simulink model "Combined"  (R2022a)
settings: Solver=FixedStepAuto  StartTime=0.0  StopTime=10.0  FixedStep=1e-3  RelTol=1e-3  EnableMultiTasking=on
undefined symbols (not defined in the file or in its folder): D0, D1, D10, D11, D12, D13, D2, D4, D5, D6, D7, D8, D9, PTA0, PTA2, PTB23, PTB9, PTC16, PTC17, PTC2, PTC3, PTC4, PTD0, PTD1, PTD2, PTD3
libraries: frdmk64flib x14
settings Model: ExtModeTrigDuration=5  Creator=anand  LastModifiedBy=anand
settings OptimizationCC: EnhancedBackFolding=on  PassReuseOutputArgsAs=Individual arguments  ZeroExternalMemoryAtStartup=off  ZeroInternalMemoryAtStartup=off  MaxStackSize=64  OptimizeBlockOrder=speed  DifferentSizesBufferReuse=on  OptimizationCustomize=off  EfficientTunableParamExpr=on
settings DebuggingCC: ParameterTunabilityLossMsg=error
settings HardwareCC: ProdBitPerPointer=32  ProdBitPerSizeT=32  ProdBitPerPtrDiffT=32  ProdLargestAtomicInteger=Long  ProdLargestAtomicFloat=Double  ProdWordSize=32  ProdHWDeviceType=ARM Compatible->ARM Cortex
settings SFSimCC: MATLABDynamicMemAlloc=off
settings RTWCC: SystemTargetFile=ert.tlc  HardwareBoard=NXP FRDM-K64F  TLCOptions="-aInlineSetEventsForThisBaseRateFcn=TLC_FALSE -aSuppressMultiTaskScheduler=TLC_FALSE  -aRateBasedStepFcn=0"  TemplateMakefile=ert_default_tmf  Toolchain=GNU Tools for ARM Embedded Processors
settings CodeAppCC: ForceParamTrailComments=on  IgnoreCustomStorageClasses=off  OperatorAnnotations=on  SimulinkDataObjDesc=on  SFDataObjDesc=on  InsertBlockDesc=on
settings ERTTargetCC: ExtModeTransport=4  ExtModeMexFile=sendToCommService

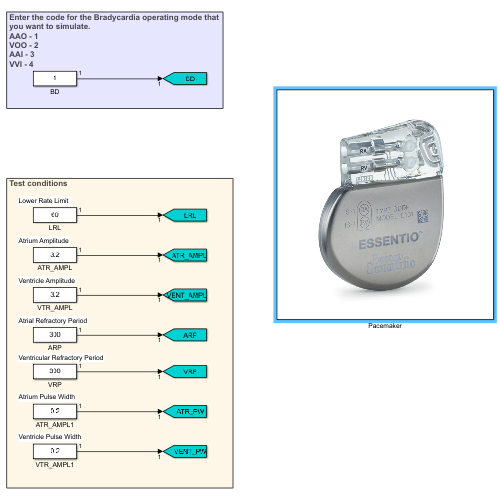
[thumbnail: Simulink's stored preview of the top-level diagram]
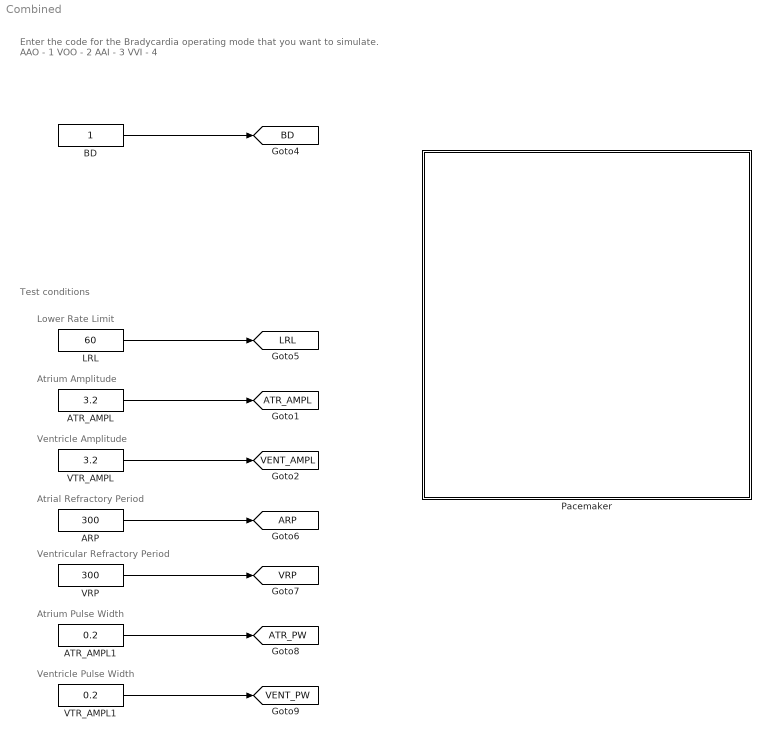
== system Combined ==
  note: Lower Rate Limit
  note: Test conditions
  note: Enter the code for the Bradycardia operating mode that
      | you want to simulate.
      | AAO - 1
      | VOO - 2
      | AAI - 3
      | VVI - 4
  note: Atrium Amplitude
  note: Ventricle Amplitude
  note: Atrial Refractory Period
  note: Ventricular Refractory Period
  note: Atrium Pulse Width
  note: Ventricle Pulse Width
  ARP : Constant  Value=300
  ATR_AMPL : Constant  Value=3.2
  ATR_AMPL1 : Constant  Value=0.2
  BD : Constant
  LRL : Constant  Value=60
  Pacemaker : Subsystem
      mask Display: image('$imagefile'); % Use "Edit Image" on toolstrip to change.
  VRP : Constant  Value=300
  VTR_AMPL : Constant  Value=3.2
  VTR_AMPL1 : Constant  Value=0.2
  tag scope: ARP=global, ATR_AMPL=global, ATR_PW=global, BD=global, LRL=global, VENT_AMPL=global, VENT_PW=global, VRP=global
  wires:
  LRL/1 -> [LRL]
  BD/1 -> [BD]
  ATR_AMPL/1 -> [ATR_AMPL]
  VTR_AMPL/1 -> [VENT_AMPL]
  ARP/1 -> [ARP]
  VRP/1 -> [VRP]
  ATR_AMPL1/1 -> [ATR_PW]
  VTR_AMPL1/1 -> [VENT_PW]

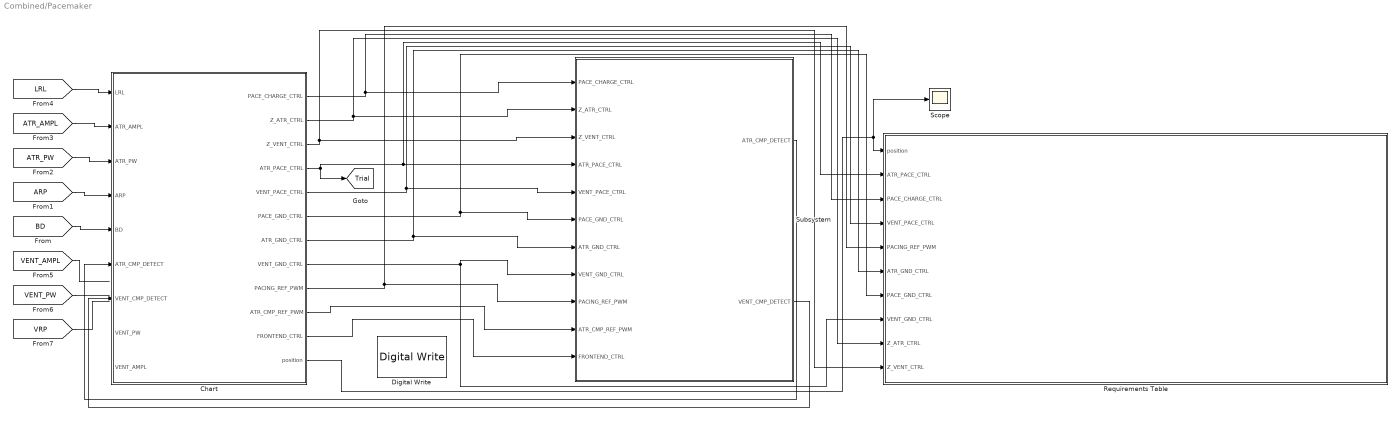
== system Combined/Pacemaker ==
  Chart : Stateflow chart  TreatAsAtomicUnit=on
  Digital Write : frdmk64flib/Digital Write  Whichpin=RED_LED
  Requirements Table : Requirements Table  TreatAsAtomicUnit=on
  Scope : Scope
  Subsystem : Subsystem
  tag scope: Trial=global
  wires:
  Chart/1(PACE_CHARGE_CTRL) -> Requirements Table/3(PACE_CHARGE_CTRL), Subsystem/1(PACE_CHARGE_CTRL)
  Chart/11(FRONTEND_CTRL) -> Subsystem/11(FRONTEND_CTRL)
  Subsystem/1(ATR_CMP_DETECT) -> Chart/6(ATR_CMP_DETECT)
  Chart/2(Z_ATR_CTRL) -> Requirements Table/9(Z_ATR_CTRL), Subsystem/2(Z_ATR_CTRL)
  Chart/6(PACE_GND_CTRL) -> Requirements Table/7(PACE_GND_CTRL), Subsystem/6(PACE_GND_CTRL)
  Chart/3(Z_VENT_CTRL) -> Requirements Table/10(Z_VENT_CTRL), Subsystem/3(Z_VENT_CTRL)
  Chart/9(PACING_REF_PWM) -> Requirements Table/5(PACING_REF_PWM), Subsystem/9(PACING_REF_PWM)
  Chart/8(VENT_GND_CTRL) -> Requirements Table/8(VENT_GND_CTRL), Subsystem/8(VENT_GND_CTRL)
  Chart/10(ATR_CMP_REF_PWM) -> Subsystem/10(ATR_CMP_REF_PWM)
  Chart/7(ATR_GND_CTRL) -> Requirements Table/6(ATR_GND_CTRL), Subsystem/7(ATR_GND_CTRL)
  Chart/5(VENT_PACE_CTRL) -> Requirements Table/4(VENT_PACE_CTRL), Subsystem/5(VENT_PACE_CTRL)
  Chart/4(ATR_PACE_CTRL) -> [Trial], Requirements Table/2(ATR_PACE_CTRL), Subsystem/4(ATR_PACE_CTRL)
  [BD] -> Chart/5(BD)
  [ATR_AMPL] -> Chart/2(ATR_AMPL)
  [ARP] -> Chart/4(ARP)
  [LRL] -> Chart/1(LRL)
  [ATR_PW] -> Chart/3(ATR_PW)
  [VENT_AMPL] -> ?
  [VENT_PW] -> ?
  [VRP] -> ?
  Subsystem/2(VENT_CMP_DETECT) -> Chart/7(VENT_CMP_DETECT)
  Chart/12(position) -> Scope/1, Requirements Table/1(position)

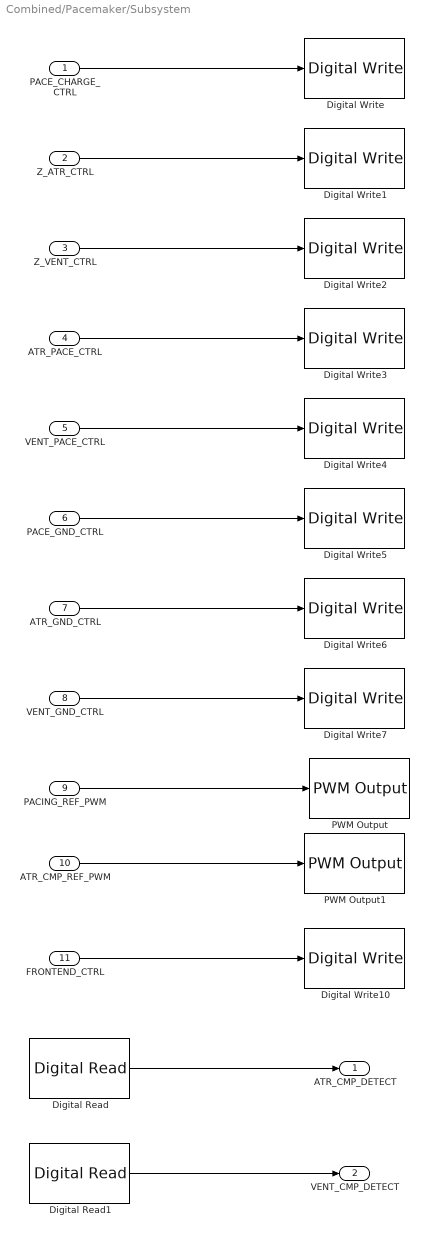
== system Combined/Pacemaker/Subsystem ==
  PACE_CHARGE_CTRL : Inport  OutDataTypeStr=boolean
  Z_ATR_CTRL : Inport  Port=2  OutDataTypeStr=boolean
  Z_VENT_CTRL : Inport  Port=3
  ATR_PACE_CTRL : Inport  Port=4
  VENT_PACE_CTRL : Inport  Port=5
  PACE_GND_CTRL : Inport  Port=6
  ATR_GND_CTRL : Inport  Port=7
  VENT_GND_CTRL : Inport  Port=8
  PACING_REF_PWM : Inport  Port=9
  ATR_CMP_REF_PWM : Inport  Port=10
  FRONTEND_CTRL : Inport  Port=11
  Digital Read : frdmk64flib/Digital Read  Whichpin=PTC16 (D0)  SampleTime=-1
  Digital Read1 : frdmk64flib/Digital Read  Whichpin=PTC17 (D1)  SampleTime=-1
  Digital Write : frdmk64flib/Digital Write  Whichpin=PTB9 (D2)
  Digital Write1 : frdmk64flib/Digital Write  Whichpin=PTB23 (D4)
  Digital Write10 : frdmk64flib/Digital Write  Whichpin=PTD1 (D13)
  Digital Write2 : frdmk64flib/Digital Write  Whichpin=PTC3 (D7)
  Digital Write3 : frdmk64flib/Digital Write  Whichpin=PTA0 (D8)
  Digital Write4 : frdmk64flib/Digital Write  Whichpin=PTC4 (D9)
  Digital Write5 : frdmk64flib/Digital Write  Whichpin=PTD0 (D10)
  Digital Write6 : frdmk64flib/Digital Write  Whichpin=PTD2 (D11)
  Digital Write7 : frdmk64flib/Digital Write  Whichpin=PTD3 (D12)
  PWM Output : frdmk64flib/PWM Output  Whichpin=PTA2 (D5)  InitialFrequency=2000  InitialDutyCycle=0
  PWM Output1 : frdmk64flib/PWM Output  Whichpin=PTC2 (D6)  InitialFrequency=2000  InitialDutyCycle=0
  ATR_CMP_DETECT : Outport  OutDataTypeStr=boolean
  VENT_CMP_DETECT : Outport  Port=2  OutDataTypeStr=boolean
  wires:
  PACE_CHARGE_CTRL/1 -> Digital Write/1
  Z_ATR_CTRL/1 -> Digital Write1/1
  Z_VENT_CTRL/1 -> Digital Write2/1
  ATR_PACE_CTRL/1 -> Digital Write3/1
  VENT_PACE_CTRL/1 -> Digital Write4/1
  PACE_GND_CTRL/1 -> Digital Write5/1
  ATR_GND_CTRL/1 -> Digital Write6/1
  VENT_GND_CTRL/1 -> Digital Write7/1
  PACING_REF_PWM/1 -> PWM Output/1
  ATR_CMP_REF_PWM/1 -> PWM Output1/1
  Digital Read/1 -> ATR_CMP_DETECT/1
  FRONTEND_CTRL/1 -> Digital Write10/1
  Digital Read1/1 -> VENT_CMP_DETECT/1

== stateflow chart Combined/Pacemaker/Requirements Table ==
  state VVI
    state CHARGING
      entry:
      %CHARGING C22
      FRONTEND_CTRL = true;
      VENT_PACE_CTRL = false;
      ATR_PACE_CTRL = false;
      PACE_CHARGE_CTRL = true;
      PACING_REF_PWM = 100*ATR_AMPL/5;
      ATR_CMP_REF_PWM = 55;
      LED = false;
    state PACE_ATR
      entry:
      PACE_CHARGE_CTRL = false;
      PACE_GND_CTRL = true;
      VENT_PACE_CTRL = false;
      VENT_GND_CTRL = false;
      Z_VENT_CTRL = false;
      Z_ATR_CTRL = false;
      ATR_GND_CTRL = false;
      ATR_PACE_CTRL = true;
    state Atrial_Refractory_Period_Post_Sensing
      LED = true;
    state DISCHARGING
      entry:
      %DISCHARGING C21
      PACE_GND_CTRL = true;
      ATR_PACE_CTRL = false;
      Z_VENT_CTRL = false;
      Z_ATR_CTRL = false;
      VENT_PACE_CTRL = false;
      VENT_GND_CTRL = false;
      ATR_GND_CTRL = true;
    (default) -> VVI.CHARGING : {delta = 0}
    VVI.CHARGING -> VVI.PACE_ATR [order 2] : after(60000/LRL-delta-ATR_PW, msec)
    VVI.CHARGING -> VVI.Atrial_Refractory_Period_Post_Sensing [order 1] : [VENT_CMP_DETECT == true]
    VVI.Atrial_Refractory_Period_Post_Sensing -> VVI.CHARGING : after(ARP,msec){delta = ARP}
    VVI.DISCHARGING -> VVI.CHARGING : after(ARP,msec){delta=ARP}
    VVI.PACE_ATR -> VVI.DISCHARGING : after(ATR_PW,msec)
  state VVI1
    state CHARGING
      entry:
      %CHARGING C22
      FRONTEND_CTRL = true;
      VENT_PACE_CTRL = false;
      ATR_PACE_CTRL = false;
      PACE_CHARGE_CTRL = true;
      PACING_REF_PWM = 100*ATR_AMPL/5;
      ATR_CMP_REF_PWM = 55;
      LED = false;
    state PACE_ATR
      entry:
      PACE_CHARGE_CTRL = false;
      PACE_GND_CTRL = true;
      VENT_PACE_CTRL = false;
      VENT_GND_CTRL = false;
      Z_VENT_CTRL = false;
      Z_ATR_CTRL = false;
      ATR_GND_CTRL = false;
      ATR_PACE_CTRL = true;
    state Atrial_Refractory_Period_Post_Sensing
      LED = true;
    state DISCHARGING
      entry:
      %DISCHARGING C21
      PACE_GND_CTRL = true;
      ATR_PACE_CTRL = false;
      Z_VENT_CTRL = false;
      Z_ATR_CTRL = false;
      VENT_PACE_CTRL = false;
      VENT_GND_CTRL = false;
      ATR_GND_CTRL = true;
    (default) -> VVI1.CHARGING : {delta = 0}
    VVI1.CHARGING -> VVI1.PACE_ATR [order 2] : after(60000/LRL-delta-ATR_PW, msec)
    VVI1.CHARGING -> VVI1.Atrial_Refractory_Period_Post_Sensing [order 1] : [VENT_CMP_DETECT == true]
    VVI1.Atrial_Refractory_Period_Post_Sensing -> VVI1.CHARGING : after(ARP,msec){delta = ARP}
    VVI1.DISCHARGING -> VVI1.CHARGING : after(ARP,msec){delta=ARP}
    VVI1.PACE_ATR -> VVI1.DISCHARGING : after(ATR_PW,msec)
  state VVI2
    state CHARGING
      entry:
      %CHARGING C22
      FRONTEND_CTRL = true;
      VENT_PACE_CTRL = false;
      ATR_PACE_CTRL = false;
      PACE_CHARGE_CTRL = true;
      PACING_REF_PWM = 100*ATR_AMPL/5;
      ATR_CMP_REF_PWM = 55;
      LED = false;
    state PACE_ATR
      entry:
      PACE_CHARGE_CTRL = false;
      PACE_GND_CTRL = true;
      VENT_PACE_CTRL = false;
      VENT_GND_CTRL = false;
      Z_VENT_CTRL = false;
      Z_ATR_CTRL = false;
      ATR_GND_CTRL = false;
      ATR_PACE_CTRL = true;
    state Atrial_Refractory_Period_Post_Sensing
      LED = true;
    state DISCHARGING
      entry:
      %DISCHARGING C21
      PACE_GND_CTRL = true;
      ATR_PACE_CTRL = false;
      Z_VENT_CTRL = false;
      Z_ATR_CTRL = false;
      VENT_PACE_CTRL = false;
      VENT_GND_CTRL = false;
      ATR_GND_CTRL = true;
    (default) -> VVI2.CHARGING : {delta = 0}
    VVI2.CHARGING -> VVI2.PACE_ATR [order 2] : after(60000/LRL-delta-ATR_PW, msec)
    VVI2.CHARGING -> VVI2.Atrial_Refractory_Period_Post_Sensing [order 1] : [VENT_CMP_DETECT == true]
    VVI2.Atrial_Refractory_Period_Post_Sensing -> VVI2.CHARGING : after(ARP,msec){delta = ARP}
    VVI2.DISCHARGING -> VVI2.CHARGING : after(ARP,msec){delta=ARP}
    VVI2.PACE_ATR -> VVI2.DISCHARGING : after(ATR_PW,msec)
  (default) -> (junction 1073742040)
  (junction 1073742040) -> (junction 1073742041) : {
      | % SF_REQ_REV_07
      | }
  (junction 1073742041) -> (junction 1073742043) : {
      | % HEADER_ASSIGNMENTS
      |
      | }
  (junction 1073742043) -> (junction 1073742045) : {
      | % START_A_4
      | }
  (junction 1073742045) -> (junction 1073742047) : {
      | }
  (junction 1073742047) -> (junction 1073742049)
  (junction 1073742049) -> (junction 1073742051) : {
      | }
  (junction 1073742051) -> (junction 1073742053) : {
      | % END_A_4
      | }
  (junction 1073742053) -> (junction 1073742055) : {
      | % START_R_1
      | }
  (junction 1073742055) -> (junction 1073742057) : {
      | }
  (junction 1073742057) -> (junction 1073742059)
  (junction 1073742059) -> (junction 1073742061) [order 1] : [(position == 1)]
  (junction 1073742059) -> (junction 1073742067) [order 2]
  (junction 1073742061) -> (junction 1073742063) : {
      | reqtable_postcondition((ATR_PACE_CTRL == false ) && (VENT_PACE_CTRL ==0) && (PACE_CHARGE_CTRL == 1 ) && (PACING_REF_PWM == 1), 'R:1');
      |
      |
      | }
  (junction 1073742063) -> (junction 1073742065) : {
      | }
  (junction 1073742065) -> (junction 1073742067)
  (junction 1073742067) -> (junction 1073742069)
  (junction 1073742069) -> (junction 1073742071) : {
      | % END_R_1
      | }
  (junction 1073742071) -> (junction 1073742073) : {
      | % START_R_7
      | }
  (junction 1073742073) -> (junction 1073742075) : {
      | }
  (junction 1073742075) -> (junction 1073742077)
  (junction 1073742077) -> (junction 1073742079) [order 1] : [(position == 2 )]
  (junction 1073742077) -> (junction 1073742085) [order 2]
  (junction 1073742079) -> (junction 1073742081) : {
      | reqtable_postcondition((PACE_CHARGE_CTRL == 0 && PACE_GND_CTRL == 1 && ATR_PACE_CTRL == 0 && ATR_GND_CTRL == 0 && Z_ATR_CTRL == 0 && Z_VENT_CTRL == 0 && VENT_GND_CTRL == 0 && VENT_PACE_CTRL ==1 ), 'R:2');
      |
      |
      | }
  (junction 1073742081) -> (junction 1073742083) : {
      | }
  (junction 1073742083) -> (junction 1073742085)
  (junction 1073742085) -> (junction 1073742087)
  (junction 1073742087) -> (junction 1073742089) : {
      | % END_R_7
      | }
  (junction 1073742089) -> (junction 1073742091) : {
      | % START_R_10
      | }
  (junction 1073742091) -> (junction 1073742093) : {
      | }
  (junction 1073742093) -> (junction 1073742095)
  (junction 1073742095) -> (junction 1073742097) [order 1] : [(position == 3 )]
  (junction 1073742095) -> (junction 1073742103) [order 2]
  (junction 1073742097) -> (junction 1073742099) : {
      | reqtable_postcondition((PACE_GND_CTRL == 1 && VENT_PACE_CTRL == 0 && Z_ATR_CTRL == 0 &&  ATR_PACE_CTRL ==0 && ATR_GND_CTRL == 0 && VENT_GND_CTRL ==1 ), 'R:3');
      |
      |
      | }
  (junction 1073742099) -> (junction 1073742101) : {
      | }
  (junction 1073742101) -> (junction 1073742103)
  (junction 1073742103) -> (junction 1073742105)
  (junction 1073742105) -> (junction 1073742107) : {
      | % END_R_10
      | }
  data: position input; ATR_PACE_CTRL input boolean; PACE_CHARGE_CTRL input boolean; VENT_PACE_CTRL input boolean; PACING_REF_PWM input double; ATR_GND_CTRL input boolean; PACE_GND_CTRL input boolean; VENT_GND_CTRL input boolean; Z_ATR_CTRL input boolean; Z_VENT_CTRL input boolean

== stateflow chart Combined/Pacemaker/Chart ==
  state AOO
    state CHARGING_DISCHARGING
      entry:
      position = 1;
      %DISCHARGING C21
      PACE_GND_CTRL = true;
      VENT_PACE_CTRL = false;
      Z_ATR_CTRL = false;
      Z_VENT_CTRL = false;
      ATR_PACE_CTRL = false;
      ATR_GND_CTRL = true;
      VENT_GND_CTRL = false;
      %CHARGING C22
      PACING_REF_PWM = 1;
      PACE_CHARGE_CTRL = true;
    state PACE_ATR
      entry:
      position =2;
      PACE_CHARGE_CTRL = false;
      PACE_GND_CTRL = true;
      ATR_PACE_CTRL = true;
      ATR_GND_CTRL = false;
      Z_ATR_CTRL = false;
      Z_VENT_CTRL = false;
      VENT_GND_CTRL = false;
      VENT_PACE_CTRL = false;
    (default) -> AOO.CHARGING_DISCHARGING
    AOO.CHARGING_DISCHARGING -> AOO.PACE_ATR : [after(60000/LRL-ATR_PW, msec)]
    AOO.PACE_ATR -> AOO.CHARGING_DISCHARGING : [after(ATR_PW,msec)]
  state VOO
    state CHARGING_DISCHARGING
      entry:
      %DISCHARGING C21
      PACE_GND_CTRL = true;
      VENT_PACE_CTRL = false;
      Z_ATR_CTRL = false;
      Z_VENT_CTRL = false;
      ATR_PACE_CTRL = false;
      ATR_GND_CTRL = false;
      VENT_GND_CTRL = true;
      %CHARGING C22
      PACING_REF_PWM = 100*VENT_AMPL/5;
      PACE_CHARGE_CTRL = true;
    state PACE_ATR
      entry:
      PACE_CHARGE_CTRL = false;
      PACE_GND_CTRL = true;
      ATR_PACE_CTRL = false;
      ATR_GND_CTRL = false;
      Z_ATR_CTRL = false;
      Z_VENT_CTRL = false;
      VENT_GND_CTRL = false;
      VENT_PACE_CTRL = true;
    (default) -> VOO.CHARGING_DISCHARGING
    VOO.CHARGING_DISCHARGING -> VOO.PACE_ATR : [after(60000/LRL-VENT_PW, msec)]
    VOO.PACE_ATR -> VOO.CHARGING_DISCHARGING : [after(VENT_PW,msec)]
  state Start
    entry:
  state AAI
    state CHARGING
      entry:
      %CHARGING C22
      FRONTEND_CTRL = true;
      VENT_PACE_CTRL = false;
      ATR_PACE_CTRL = false;
      PACE_CHARGE_CTRL = true;
      PACING_REF_PWM = 90;
      ATR_CMP_REF_PWM = 90;
    state PACE_ATR
      entry:
      PACE_CHARGE_CTRL = false;
      PACE_GND_CTRL = true;
      VENT_PACE_CTRL = false;
      VENT_GND_CTRL = false;
      Z_VENT_CTRL = false;
      Z_ATR_CTRL = false;
      ATR_GND_CTRL = false;
      ATR_PACE_CTRL = true;
    state Atrial_Refractory_Period_Post_Sensing
      entry:
    state DISCHARGING
      entry:
      %DISCHARGING C21
      PACE_GND_CTRL = true;
      ATR_PACE_CTRL = false;
      Z_VENT_CTRL = false;
      Z_ATR_CTRL = false;
      VENT_PACE_CTRL = false;
      VENT_GND_CTRL = false;
      ATR_GND_CTRL = true;
    (default) -> AAI.CHARGING : {delta = 0; sensing = 0}
    AAI.CHARGING -> AAI.PACE_ATR [order 2] : [after(60000/LRL-delta-ATR_PW, msec)]
    AAI.CHARGING -> AAI.Atrial_Refractory_Period_Post_Sensing [order 1] : [ATR_CMP_DETECT == true]
    AAI.Atrial_Refractory_Period_Post_Sensing -> AAI.CHARGING : [after(ARP,msec)]{delta = ARP; sensing = 1}
    (junction 130) -> AAI.CHARGING : [after(ARP,msec)]{delta=0; sensing = 0}
    (junction 131) -> AAI.CHARGING : [after(ARP,msec)]{delta=ARP}
    AAI.PACE_ATR -> AAI.DISCHARGING : [after(ATR_PW,msec)]
    AAI.DISCHARGING -> (junction 131) [order 1] : [sensing == 0]
    AAI.DISCHARGING -> (junction 130) [order 2] : [sensing == 1]
  state VVI
    state CHARGING
      entry:
      %CHARGING C22
      FRONTEND_CTRL = true;
      VENT_PACE_CTRL = false;
      ATR_PACE_CTRL = false;
      PACE_CHARGE_CTRL = true;
      PACING_REF_PWM = 100*ATR_AMPL/5;
      ATR_CMP_REF_PWM = 55;
    state PACE_ATR
      entry:
      PACE_CHARGE_CTRL = false;
      PACE_GND_CTRL = true;
      VENT_PACE_CTRL = false;
      VENT_GND_CTRL = false;
      Z_VENT_CTRL = false;
      Z_ATR_CTRL = false;
      ATR_GND_CTRL = false;
      ATR_PACE_CTRL = true;
    state Atrial_Refractory_Period_Post_Sensing
    state DISCHARGING
      entry:
      %DISCHARGING C21
      PACE_GND_CTRL = true;
      ATR_PACE_CTRL = false;
      Z_VENT_CTRL = false;
      Z_ATR_CTRL = false;
      VENT_PACE_CTRL = false;
      VENT_GND_CTRL = false;
      ATR_GND_CTRL = true;
    (default) -> VVI.CHARGING : {delta = 0}
    VVI.CHARGING -> VVI.PACE_ATR [order 2] : after(60000/LRL-delta-ATR_PW, msec)
    VVI.CHARGING -> VVI.Atrial_Refractory_Period_Post_Sensing [order 1] : [VENT_CMP_DETECT == true]
    VVI.Atrial_Refractory_Period_Post_Sensing -> VVI.CHARGING : after(ARP,msec){delta = ARP}
    VVI.DISCHARGING -> VVI.CHARGING : after(ARP,msec){delta=ARP}
    VVI.PACE_ATR -> VVI.DISCHARGING : after(ATR_PW,msec)
  Start -> AOO [order 1] : [BD == 1]
  Start -> VOO [order 2] : [BD == 2]
  (default) -> Start
  Start -> AAI [order 3] : [BD == 3]
  Start -> VVI [order 4] : [BD == 4]
  data: LRL input size=[1]; ATR_AMPL input size=[1]; ATR_PW input size=[1]; PACE_CHARGE_CTRL output boolean; Z_ATR_CTRL output; Z_VENT_CTRL output; ATR_PACE_CTRL output; VENT_PACE_CTRL output; PACE_GND_CTRL output; ATR_GND_CTRL output; VENT_GND_CTRL output; PACING_REF_PWM output; ARP input size=[1]; ATR_CMP_REF_PWM output; delta local double; FRONTEND_CTRL output; BD input size=[1]; ATR_CMP_DETECT input boolean size=[1,1]; VENT_CMP_DETECT input boolean size=[1,1]; sensing local; VENT_PW input size=[1]; VENT_AMPL input size=[1]; position output
